simulink model "narwhale_3dof_dynamics_func"  (R2021b)
settings: Solver=VariableStepAuto  StartTime=0.0  StopTime=5  RelTol=1e-3
undefined symbols (not defined in the file or in its folder): X, Y, Z
libraries: sm_lib x20, nesl_utility x10
(part 2 of 2)

== matlab function narwhale_3dof_dynamics_func/NarWhale/MATLAB Function ==
  data: q1d input; ut output; q1v input; q1a input; q2d input; q2v input; q2a input; q3d input; q3v input; q3a input
function ut = fcn(q1d,q1v,q1a,q2d,q2v,q2a,q3d,q3v,q3a)

m1 = 3.0358
m2 = 2.0778
m3 = 1.4388
I1 = [0.00971694169       -0.00064648471      -0.01364762489;
      -0.00064648471        0.01128154665     -0.00136042243;
      -0.01364762489    -0.00136042243       0.01196416148];
I2 = [0.00247391072       -0.00003538205         -0.00217523776;
      -0.00003538205         0.03115417518       0.000038745;
      -0.00217523776       0.000038745         0.029417341];
I3 = [0.0016       0.00001724909   -0.00032435212;
      0.00001724909   0.0174       0.00000416776;
      -0.00032435212    0.00000416776       0.0164];

m = [m1 m2 m3]
I = cat(3,I1,I2,I3)
q = [q1d;q2d;q3d];
qd = [q1v;q2v ;q3v];
qdd = [q1a;q2a;q3a];
rho = [1;1;1];
%%
% parameters
    cm1 = [-43.29; -2.02; -88.16]./1000.0;
    cm2 = [162; -0.02; 8.59]./1000.0;
    cm3 = [-175.56; 0.06; -6.33]./1000.0;
    cm=cat(3,cm1,cm2,cm3);
    %find m
    Mt =zeros(3,3);
    Ct =zeros(3,3);
    Gt =zeros(3,1);
    ut =zeros(3,1);
    M = zeros(3,3,3);
    Hcm = zeros(4,4,3);
    Jwc = zeros(3,3,3);
    Jvc = zeros(3,3,3);
    % forwardkinematics
    h1= 275.99/1000.0; % lasted
    h2= 380.0/1000.0;
    l1= 20.0/1000.0;
    l2= 380.0/1000.0;
    l3= 268.23/1000.0;
    DH =[0   0   h1   0;
        l1 pi/2  0  pi/2;
        h2  0    0  -pi/2];
    
    Hne=[1 0  0  l2 ;
         0 1  0  0; 
         0 0  1  0;
         0 0  0  1];
    H1c1 = [1 0 0 cm1(1);
       0 1 0  cm1(2);
       0 0 1  cm1(3);
       0 0 0     1];
    H2c2 = [1 0 0 cm2(1);
            0 1 0 cm2(2);
            0 0 1 cm2(3);
            0 0 0    1];
    H3c3 = [1 0 0 cm3(1);
            0 1 0 cm3(2);
            0 0 1 cm3(3);
            0 0 0    1];
    m1 = m(1);
    m2 = m(2);
    m3 = m(3);
    g = 9.80665;

    q1 =q(1);
    q2 =q(2);
    q3 =q(3);
    q1d = qd(1);
    q2d = qd(2);
    q3d = qd(3);
    q1dd = qdd(1);
    q2dd = qdd(2);
    q3dd = qdd(3);
    H = forwardKinematics(q(1:3),rho,DH,Hne);
    Hcm(:,:,1) = H(:,:,1)*H1c1;
    Hcm(:,:,2) = H(:,:,2)*H2c2;
    Hcm(:,:,3) = H(:,:,3)*H3c3;
    S =@(P) [ 0   -P(3)  P(2);
              P(3)  0    -P(1);
             -P(2)  P(1)   0];
        
%         Jv_c1 = J(4:6,:,1)+S(H(1:3,1:3,1)*cm1).' * J(1:3,:,1);
%         Jv_c2 = J(4:6,:,2)+S(H(1:3,1:3,2)*cm2).' * J(1:3,:,2);
%         Jv_c3 = J(4:6,:,3)+S(H(1:3,1:3,3)*cm3).' * J(1:3,:,3);
    %Jacobian
    Jwc(:,:,1) = [0, 0, 0;
              0, 0, 0;
              1, 0, 0];
    Jwc(:,:,2) =[0,  sin(q1), 0;
             0, -cos(q1), 0;
             1,        0, 0];
    Jwc(:,:,3) =[0,  sin(q1),  sin(q1);
             0, -cos(q1), -cos(q1);
             1,        0,        0];
    Jvc(:,:,1) =[- cm1(2)*cos(q1) - cm1(1)*sin(q1), 0, 0;
               cm1(1)*cos(q1) - cm1(2)*sin(q1), 0, 0;
                                         0, 0, 0];
    Jvc(:,:,2) =[cm2(3)*cos(q1) - l1*sin(q1) + cm2(2)*cos(q2)*sin(q1) + cm2(1)*sin(q1)*sin(q2), -cos(q1)*(cm2(1)*cos(q2) - cm2(2)*sin(q2)), 0;
             l1*cos(q1) + cm2(3)*sin(q1) - cm2(2)*cos(q1)*cos(q2) - cm2(1)*cos(q1)*sin(q2), -sin(q1)*(cm2(1)*cos(q2) - cm2(2)*sin(q2)), 0;
                                                                                   0,          - cm2(2)*cos(q2) - cm2(1)*sin(q2), 0]
    Jvc(:,:,3) =[cm3(3)*cos(q1) - l1*sin(q1) - cm3(1)*cos(q2 + q3)*sin(q1) + cm3(2)*sin(q2 + q3)*sin(q1) + h2*sin(q1)*sin(q2), -cos(q1)*(cm3(2)*cos(q2 + q3) + cm3(1)*sin(q2 + q3) + h2*cos(q2)), -cos(q1)*(cm3(2)*cos(q2 + q3) + cm3(1)*sin(q2 + q3));
             l1*cos(q1) + cm3(3)*sin(q1) + cm3(1)*cos(q2 + q3)*cos(q1) - cm3(2)*sin(q2 + q3)*cos(q1) - h2*cos(q1)*sin(q2), -sin(q1)*(cm3(2)*cos(q2 + q3) + cm3(1)*sin(q2 + q3) + h2*cos(q2)), -sin(q1)*(cm3(2)*cos(q2 + q3) + cm3(1)*sin(q2 + q3));
                                                                                                                       0,            cm3(1)*cos(q2 + q3) - cm3(2)*sin(q2 + q3) - h2*sin(q2),            cm3(1)*cos(q2 + q3) - cm3(2)*sin(q2 + q3)];
 
    for j = 1:numel(rho)
            M(:,:,j) = (m(j)*(Jvc(:,:,j)')*Jvc(:,:,j)) + ((Jwc(:,:,j)')*Hcm(1:3,1:3,j)*I(:,:,j)*Hcm(1:3,1:3,j)'*Jwc(1:3,:,j));
    end
        sigmaM = M(:,:,1) + M(:,:,2) + M(:,:,3);
        Mt(:,:)=sigmaM;
        
        C = [0.5000*q3d*(cos(q2 + q3)*(I(2,1,3)*cos(q2 + q3) + I(1,1,3)*sin(q2 + q3)) + cos(q2 + q3)*(I(1,2,3)*cos(q2 + q3) - I(2,2,3)*sin(q2 + q3)) + sin(q2 + q3)*(I(1,1,3)*cos(q2 + q3) - I(2,1,3)*sin(q2 + q3)) - sin(q2 + q3)*(I(2,2,3)*cos(q2 + q3) + I(1,2,3)*sin(q2 + q3)) - 2*m3*(cm3(2)*cos(q2 + q3)*cos(q1) + cm3(1)*sin(q2 + q3)*cos(q1))*(l1*cos(q1) + cm3(3)*sin(q1) + cm3(1)*cos(q2 + q3)*cos(q1) - cm3(2)*sin(q2 + q3)*cos(q1) - h2*cos(q1)*sin(q2)) + 2*m3*(cm3(2)*cos(q2 + q3)*sin(q1) + cm3(1)*sin(q2 + q3)*sin(q1))*(cm3(3)*cos(q1) - l1*sin(q1) - cm3(1)*cos(q2 + q3)*sin(q1) + cm3(2)*sin(q2 + q3)*sin(q1) + h2*sin(q1)*sin(q2))) + 0.5000*q2d*(cos(q2 + q3)*(I(2,1,3)*cos(q2 + q3) + I(1,1,3)*sin(q2 + q3)) + cos(q2 + q3)*(I(1,2,3)*cos(q2 + q3) - I(2,2,3)*sin(q2 + q3)) + sin(q2 + q3)*(I(1,1,3)*cos(q2 + q3) - I(2,1,3)*sin(q2 + q3)) - sin(q2 + q3)*(I(2,2,3)*cos(q2 + q3) + I(1,2,3)*sin(q2 + q3)) - cos(q2)*(I(2,1,2)*cos(q2) + I(1,1,2)*sin(q2)) - cos(q2)*(I(1,2,2)*cos(q2) - I(2,2,2)*sin(q2)) - sin(q2)*(I(1,1,2)*cos(q2) - I(2,1,2)*sin(q2)) + sin(q2)*(I(2,2,2)*cos(q2) + I(1,2,2)*sin(q2)) + 2*m3*(cm3(2)*cos(q2 + q3)*sin(q1) + cm3(1)*sin(q2 + q3)*sin(q1) + h2*cos(q2)*sin(q1))*(cm3(3)*cos(q1) - l1*sin(q1) - cm3(1)*cos(q2 + q3)*sin(q1) + cm3(2)*sin(q2 + q3)*sin(q1) + h2*sin(q1)*sin(q2)) - 2*m2*(cm2(1)*cos(q1)*cos(q2) - cm2(2)*cos(q1)*sin(q2))*(l1*cos(q1) + cm2(3)*sin(q1) - cm2(2)*cos(q1)*cos(q2) - cm2(1)*cos(q1)*sin(q2)) - 2*m3*(cm3(2)*cos(q2 + q3)*cos(q1) + cm3(1)*sin(q2 + q3)*cos(q1) + h2*cos(q1)*cos(q2))*(l1*cos(q1) + cm3(3)*sin(q1) + cm3(1)*cos(q2 + q3)*cos(q1) - cm3(2)*sin(q2 + q3)*cos(q1) - h2*cos(q1)*sin(q2)) + 2*m2*(cm2(1)*cos(q2)*sin(q1) - cm2(2)*sin(q1)*sin(q2))*(cm2(3)*cos(q1) - l1*sin(q1) + cm2(2)*cos(q2)*sin(q1) + cm2(1)*sin(q1)*sin(q2))), 0.5000*q1d*(cos(q2 + q3)*(I(2,1,3)*cos(q2 + q3) + I(1,1,3)*sin(q2 + q3)) + cos(q2 + q3)*(I(1,2,3)*cos(q2 + q3) - I(2,2,3)*sin(q2 + q3)) + sin(q2 + q3)*(I(1,1,3)*cos(q2 + q3) - I(2,1,3)*sin(q2 + q3)) - sin(q2 + q3)*(I(2,2,3)*cos(q2 + q3) + I(1,2,3)*sin(q2 + q3)) - cos(q2)*(I(2,1,2)*cos(q2) + I(1,1,2)*sin(q2)) - cos(q2)*(I(1,2,2)*cos(q2) - I(2,2,2)*sin(q2)) - sin(q2)*(I(1,1,2)*cos(q2) - I(2,1,2)*sin(q2)) + sin(q2)*(I(2,2,2)*cos(q2) + I(1,2,2)*sin(q2)) + 2*m3*(cm3(2)*cos(q2 + q3)*sin(q1) + cm3(1)*sin(q2 + q3)*sin(q1) + h2*cos(q2)*sin(q1))*(cm3(3)*cos(q1) - l1*sin(q1) - cm3(1)*cos(q2 + q3)*sin(q1) + cm3(2)*sin(q2 + q3)*sin(q1) + h2*sin(q1)*sin(q2)) - 2*m2*(cm2(1)*cos(q1)*cos(q2) - cm2(2)*cos(q1)*sin(q2))*(l1*cos(q1) + cm2(3)*sin(q1) - cm2(2)*cos(q1)*cos(q2) - cm2(1)*cos(q1)*sin(q2)) - 2*m3*(cm3(2)*cos(q2 + q3)*cos(q1) + cm3(1)*sin(q2 + q3)*cos(q1) + h2*cos(q1)*cos(q2))*(l1*cos(q1) + cm3(3)*sin(q1) + cm3(1)*cos(q2 + q3)*cos(q1) - cm3(2)*sin(q2 + q3)*cos(q1) - h2*cos(q1)*sin(q2)) + 2*m2*(cm2(1)*cos(q2)*sin(q1) - cm2(2)*sin(q1)*sin(q2))*(cm2(3)*cos(q1) - l1*sin(q1) + cm2(2)*cos(q2)*sin(q1) + cm2(1)*sin(q1)*sin(q2))) - 0.5000*q3d*(2*sin(q1)*(cos(q2 + q3)*cos(q1)*(I(2,2,3)*cos(q2 + q3) + I(1,2,3)*sin(q2 + q3)) - cos(q2 + q3)*cos(q1)*(I(1,1,3)*cos(q2 + q3) - I(2,1,3)*sin(q2 + q3)) - sin(q1)*(I(1,3,3)*cos(q2 + q3) - I(2,3,3)*sin(q2 + q3)) + sin(q2 + q3)*cos(q1)*(I(2,1,3)*cos(q2 + q3) + I(1,1,3)*sin(q2 + q3)) + sin(q2 + q3)*cos(q1)*(I(1,2,3)*cos(q2 + q3) - I(2,2,3)*sin(q2 + q3))) - 2*cos(q1)*(cos(q1)*(I(1,3,3)*cos(q2 + q3) - I(2,3,3)*sin(q2 + q3)) + sin(q2 + q3)*sin(q1)*(I(2,1,3)*cos(q2 + q3) + I(1,1,3)*sin(q2 + q3)) + sin(q2 + q3)*sin(q1)*(I(1,2,3)*cos(q2 + q3) - I(2,2,3)*sin(q2 + q3)) - cos(q2 + q3)*sin(q1)*(I(1,1,3)*cos(q2 + q3) - I(2,1,3)*sin(q2 + q3)) + cos(q2 + q3)*sin(q1)*(I(2,2,3)*cos(q2 + q3) + I(1,2,3)*sin(q2 + q3))) - m3*sin(q1)*(cm3(2)*cos(q2 + q3) + cm3(1)*sin(q2 + q3))*(cm3(2)*cos(q2 + q3)*cos(q1) + cm3(1)*sin(q2 + q3)*cos(q1) + h2*cos(q1)*cos(q2)) + m3*cos(q1)*(cm3(2)*cos(q2 + q3) + cm3(1)*sin(q2 + q3))*(cm3(2)*cos(q2 + q3)*sin(q1) + cm3(1)*sin(q2 + q3)*sin(q1) + h2*cos(q2)*sin(q1)) - m3*sin(q1)*(cm3(2)*cos(q2 + q3)*cos(q1) + cm3(1)*sin(q2 + q3)*cos(q1))*(cm3(2)*cos(q2 + q3) + cm3(1)*sin(q2 + q3) + h2*cos(q2)) + m3*cos(q1)*(cm3(2)*cos(q2 + q3)*sin(q1) + cm3(1)*sin(q2 + q3)*sin(q1))*(cm3(2)*cos(q2 + q3) + cm3(1)*sin(q2 + q3) + h2*cos(q2)) + 2*m3*sin(q1)*(cm3(1)*cos(q2 + q3) - cm3(2)*sin(q2 + q3))*(l1*cos(q1) + cm3(3)*sin(q1) + cm3(1)*cos(q2 + q3)*cos(q1) - cm3(2)*sin(q2 + q3)*cos(q1) - h2*cos(q1)*sin(q2)) + 2*m3*cos(q1)*(cm3(1)*cos(q2 + q3) - cm3(2)*sin(q2 + q3))*(cm3(3)*cos(q1) - l1*sin(q1) - cm3(1)*cos(q2 + q3)*sin(q1) + cm3(2)*sin(q2 + q3)*sin(q1) + h2*sin(q1)*sin(q2))) + 0.5000*q2d*(2*sin(q1)*(cos(q1)*cos(q2)*(I(2,2,2)*cos(q2) + I(1,2,2)*sin(q2)) - cos(q1)*cos(q2)*(I(1,1,2)*cos(q2) - I(2,1,2)*sin(q2)) - sin(q1)*(I(2,3,2)*cos(q2) + I(1,3,2)*sin(q2)) + cos(q1)*sin(q2)*(I(2,1,2)*cos(q2) + I(1,1,2)*sin(q2)) + cos(q1)*sin(q2)*(I(1,2,2)*cos(q2) - I(2,2,2)*sin(q2))) - 2*cos(q1)*(cos(q1)*(I(2,3,2)*cos(q2) + I(1,3,2)*sin(q2)) - cos(q2)*sin(q1)*(I(1,1,2)*cos(q2) - I(2,1,2)*sin(q2)) + cos(q2)*sin(q1)*(I(2,2,2)*cos(q2) + I(1,2,2)*sin(q2)) + sin(q1)*sin(q2)*(I(2,1,2)*cos(q2) + I(1,1,2)*sin(q2)) + sin(q1)*sin(q2)*(I(1,2,2)*cos(q2) - I(2,2,2)*sin(q2))) - 2*sin(q1)*(cos(q2 + q3)*cos(q1)*(I(2,2,3)*cos(q2 + q3) + I(1,2,3)*sin(q2 + q3)) - cos(q2 + q3)*cos(q1)*(I(1,1,3)*cos(q2 + q3) - I(2,1,3)*sin(q2 + q3)) - sin(q1)*(I(1,3,3)*cos(q2 + q3) - I(2,3,3)*sin(q2 + q3)) + sin(q2 + q3)*cos(q1)*(I(2,1,3)*cos(q2 + q3) + I(1,1,3)*sin(q2 + q3)) + sin(q2 + q3)*cos(q1)*(I(1,2,3)*cos(q2 + q3) - I(2,2,3)*sin(q2 + q3))) + 2*cos(q1)*(cos(q1)*(I(1,3,3)*cos(q2 + q3) - I(2,3,3)*sin(q2 + q3)) + sin(q2 + q3)*sin(q1)*(I(2,1,3)*cos(q2 + q3) + I(1,1,3)*sin(q2 + q3)) + sin(q2 + q3)*sin(q1)*(I(1,2,3)*cos(q2 + q3) - I(2,2,3)*sin(q2 + q3)) - cos(q2 + q3)*sin(q1)*(I(1,1,3)*cos(q2 + q3) - I(2,1,3)*sin(q2 + q3)) + cos(q2 + q3)*sin(q1)*(I(2,2,3)*cos(q2 + q3) + I(1,2,3)*sin(q2 + q3))) - 2*m3*cos(q1)*(cm3(2)*cos(q2 + q3)*sin(q1) + cm3(1)*sin(q2 + q3)*sin(q1) + h2*cos(q2)*sin(q1))*(cm3(2)*cos(q2 + q3) + cm3(1)*sin(q2 + q3) + h2*cos(q2)) + 2*m3*sin(q1)*(cm3(2)*sin(q2 + q3) - cm3(1)*cos(q2 + q3) + h2*sin(q2))*(l1*cos(q1) + cm3(3)*sin(q1) + cm3(1)*cos(q2 + q3)*cos(q1) - cm3(2)*sin(q2 + q3)*cos(q1) - h2*cos(q1)*sin(q2)) + 2*m3*cos(q1)*(cm3(2)*sin(q2 + q3) - cm3(1)*cos(q2 + q3) + h2*sin(q2))*(cm3(3)*cos(q1) - l1*sin(q1) - cm3(1)*cos(q2 + q3)*sin(q1) + cm3(2)*sin(q2 + q3)*sin(q1) + h2*sin(q1)*sin(q2)) + 2*m2*sin(q1)*(cm2(1)*cos(q1)*cos(q2) - cm2(2)*cos(q1)*sin(q2))*(cm2(1)*cos(q2) - cm2(2)*sin(q2)) - 2*m2*cos(q1)*(cm2(1)*cos(q2)*sin(q1) - cm2(2)*sin(q1)*sin(q2))*(cm2(1)*cos(q2) - cm2(2)*sin(q2)) + 2*m2*sin(q1)*(cm2(2)*cos(q2) + cm2(1)*sin(q2))*(l1*cos(q1) + cm2(3)*sin(q1) - cm2(2)*cos(q1)*cos(q2) - cm2(1)*cos(q1)*sin(q2)) + 2*m3*sin(q1)*(cm3(2)*cos(q2 + q3)*cos(q1) + cm3(1)*sin(q2 + q3)*cos(q1) + h2*cos(q1)*cos(q2))*(cm3(2)*cos(q2 + q3) + cm3(1)*sin(q2 + q3) + h2*cos(q2)) + 2*m2*cos(q1)*(cm2(2)*cos(q2) + cm2(1)*sin(q2))*(cm2(3)*cos(q1) - l1*sin(q1) + cm2(2)*cos(q2)*sin(q1) + cm2(1)*sin(q1)*sin(q2))), 0.5000*q1d*(cos(q2 + q3)*(I(2,1,3)*cos(q2 + q3) + I(1,1,3)*sin(q2 + q3)) + cos(q2 + q3)*(I(1,2,3)*cos(q2 + q3) - I(2,2,3)*sin(q2 + q3)) + sin(q2 + q3)*(I(1,1,3)*cos(q2 + q3) - I(2,1,3)*sin(q2 + q3)) - sin(q2 + q3)*(I(2,2,3)*cos(q2 + q3) + I(1,2,3)*sin(q2 + q3)) - 2*m3*(cm3(2)*cos(q2 + q3)*cos(q1) + cm3(1)*sin(q2 + q3)*cos(q1))*(l1*cos(q1) + cm3(3)*sin(q1) + cm3(1)*cos(q2 + q3)*cos(q1) - cm3(2)*sin(q2 + q3)*cos(q1) - h2*cos(q1)*sin(q2)) + 2*m3*(cm3(2)*cos(q2 + q3)*sin(q1) + cm3(1)*sin(q2 + q3)*sin(q1))*(cm3(3)*cos(q1) - l1*sin(q1) - cm3(1)*cos(q2 + q3)*sin(q1) + cm3(2)*sin(q2 + q3)*sin(q1) + h2*sin(q1)*sin(q2))) - 0.5000*q2d*(2*sin(q1)*(cos(q2 + q3)*cos(q1)*(I(2,2,3)*cos(q2 + q3) + I(1,2,3)*sin(q2 + q3)) - cos(q2 + q3)*cos(q1)*(I(1,1,3)*cos(q2 + q3) - I(2,1,3)*sin(q2 + q3)) - sin(q1)*(I(1,3,3)*cos(q2 + q3) - I(2,3,3)*sin(q2 + q3)) + sin(q2 + q3)*cos(q1)*(I(2,1,3)*cos(q2 + q3) + I(1,1,3)*sin(q2 + q3)) + sin(q2 + q3)*cos(q1)*(I(1,2,3)*cos(q2 + q3) - I(2,2,3)*sin(q2 + q3))) - 2*cos(q1)*(cos(q1)*(I(1,3,3)*cos(q2 + q3) - I(2,3,3)*sin(q2 + q3)) + sin(q2 + q3)*sin(q1)*(I(2,1,3)*cos(q2 + q3) + I(1,1,3)*sin(q2 + q3)) + sin(q2 + q3)*sin(q1)*(I(1,2,3)*cos(q2 + q3) - I(2,2,3)*sin(q2 + q3)) - cos(q2 + q3)*sin(q1)*(I(1,1,3)*cos(q2 + q3) - I(2,1,3)*sin(q2 + q3)) + cos(q2 + q3)*sin(q1)*(I(2,2,3)*cos(q2 + q3) + I(1,2,3)*sin(q2 + q3))) - m3*sin(q1)*(cm3(2)*cos(q2 + q3) + cm3(1)*sin(q2 + q3))*(cm3(2)*cos(q2 + q3)*cos(q1) + cm3(1)*sin(q2 + q3)*cos(q1) + h2*cos(q1)*cos(q2)) + m3*cos(q1)*(cm3(2)*cos(q2 + q3) + cm3(1)*sin(q2 + q3))*(cm3(2)*cos(q2 + q3)*sin(q1) + cm3(1)*sin(q2 + q3)*sin(q1) + h2*cos(q2)*sin(q1)) - m3*sin(q1)*(cm3(2)*cos(q2 + q3)*cos(q1) + cm3(1)*sin(q2 + q3)*cos(q1))*(cm3(2)*cos(q2 + q3) + cm3(1)*sin(q2 + q3) + h2*cos(q2)) + m3*cos(q1)*(cm3(2)*cos(q2 + q3)*sin(q1) + cm3(1)*sin(q2 + q3)*sin(q1))*(cm3(2)*cos(q2 + q3) + cm3(1)*sin(q2 + q3) + h2*cos(q2)) + 2*m3*sin(q1)*(cm3(1)*cos(q2 + q3) - cm3(2)*sin(q2 + q3))*(l1*cos(q1) + cm3(3)*sin(q1) + cm3(1)*cos(q2 + q3)*cos(q1) - cm3(2)*sin(q2 + q3)*cos(q1) - h2*cos(q1)*sin(q2)) + 2*m3*cos(q1)*(cm3(1)*cos(q2 + q3) - cm3(2)*sin(q2 + q3))*(cm3(3)*cos(q1) - l1*sin(q1) - cm3(1)*cos(q2 + q3)*sin(q1) + cm3(2)*sin(q2 + q3)*sin(q1) + h2*sin(q1)*sin(q2))) - 0.5000*q3d*(2*sin(q1)*(cos(q2 + q3)*cos(q1)*(I(2,2,3)*cos(q2 + q3) + I(1,2,3)*sin(q2 + q3)) - cos(q2 + q3)*cos(q1)*(I(1,1,3)*cos(q2 + q3) - I(2,1,3)*sin(q2 + q3)) - sin(q1)*(I(1,3,3)*cos(q2 + q3) - I(2,3,3)*sin(q2 + q3)) + sin(q2 + q3)*cos(q1)*(I(2,1,3)*cos(q2 + q3) + I(1,1,3)*sin(q2 + q3)) + sin(q2 + q3)*cos(q1)*(I(1,2,3)*cos(q2 + q3) - I(2,2,3)*sin(q2 + q3))) - 2*cos(q1)*(cos(q1)*(I(1,3,3)*cos(q2 + q3) - I(2,3,3)*sin(q2 + q3)) + sin(q2 + q3)*sin(q1)*(I(2,1,3)*cos(q2 + q3) + I(1,1,3)*sin(q2 + q3)) + sin(q2 + q3)*sin(q1)*(I(1,2,3)*cos(q2 + q3) - I(2,2,3)*sin(q2 + q3)) - cos(q2 + q3)*sin(q1)*(I(1,1,3)*cos(q2 + q3) - I(2,1,3)*sin(q2 + q3)) + cos(q2 + q3)*sin(q1)*(I(2,2,3)*cos(q2 + q3) + I(1,2,3)*sin(q2 + q3))) + 2*m3*sin(q1)*(cm3(1)*cos(q2 + q3) - cm3(2)*sin(q2 + q3))*(l1*cos(q1) + cm3(3)*sin(q1) + cm3(1)*cos(q2 + q3)*cos(q1) - cm3(2)*sin(q2 + q3)*cos(q1) - h2*cos(q1)*sin(q2)) + 2*m3*cos(q1)*(cm3(1)*cos(q2 + q3) - cm3(2)*sin(q2 + q3))*(cm3(3)*cos(q1) - l1*sin(q1) - cm3(1)*cos(q2 + q3)*sin(q1) + cm3(2)*sin(q2 + q3)*sin(q1) + h2*sin(q1)*sin(q2)) - 2*m3*sin(q1)*(cm3(2)*cos(q2 + q3) + cm3(1)*sin(q2 + q3))*(cm3(2)*cos(q2 + q3)*cos(q1) + cm3(1)*sin(q2 + q3)*cos(q1)) + 2*m3*cos(q1)*(cm3(2)*cos(q2 + q3)*sin(q1) + cm3(1)*sin(q2 + q3)*sin(q1))*(cm3(2)*cos(q2 + q3) + cm3(1)*sin(q2 + q3)));
                                                          - 0.5000*q1d*(cos(q2 + q3)*(I(2,1,3)*cos(q2 + q3) + I(1,1,3)*sin(q2 + q3)) + cos(q2 + q3)*(I(1,2,3)*cos(q2 + q3) - I(2,2,3)*sin(q2 + q3)) + sin(q2 + q3)*(I(1,1,3)*cos(q2 + q3) - I(2,1,3)*sin(q2 + q3)) - sin(q2 + q3)*(I(2,2,3)*cos(q2 + q3) + I(1,2,3)*sin(q2 + q3)) - cos(q2)*(I(2,1,2)*cos(q2) + I(1,1,2)*sin(q2)) - cos(q2)*(I(1,2,2)*cos(q2) - I(2,2,2)*sin(q2)) - sin(q2)*(I(1,1,2)*cos(q2) - I(2,1,2)*sin(q2)) + sin(q2)*(I(2,2,2)*cos(q2) + I(1,2,2)*sin(q2)) + 2*m3*(cm3(2)*cos(q2 + q3)*sin(q1) + cm3(1)*sin(q2 + q3)*sin(q1) + h2*cos(q2)*sin(q1))*(cm3(3)*cos(q1) - l1*sin(q1) - cm3(1)*cos(q2 + q3)*sin(q1) + cm3(2)*sin(q2 + q3)*sin(q1) + h2*sin(q1)*sin(q2)) - 2*m2*(cm2(1)*cos(q1)*cos(q2) - cm2(2)*cos(q1)*sin(q2))*(l1*cos(q1) + cm2(3)*sin(q1) - cm2(2)*cos(q1)*cos(q2) - cm2(1)*cos(q1)*sin(q2)) - 2*m3*(cm3(2)*cos(q2 + q3)*cos(q1) + cm3(1)*sin(q2 + q3)*cos(q1) + h2*cos(q1)*cos(q2))*(l1*cos(q1) + cm3(3)*sin(q1) + cm3(1)*cos(q2 + q3)*cos(q1) - cm3(2)*sin(q2 + q3)*cos(q1) - h2*cos(q1)*sin(q2)) + 2*m2*(cm2(1)*cos(q2)*sin(q1) - cm2(2)*sin(q1)*sin(q2))*(cm2(3)*cos(q1) - l1*sin(q1) + cm2(2)*cos(q2)*sin(q1) + cm2(1)*sin(q1)*sin(q2))) - 0.5000*q3d*(m3*sin(q1)*(cm3(2)*cos(q2 + q3) + cm3(1)*sin(q2 + q3))*(cm3(2)*cos(q2 + q3)*cos(q1) + cm3(1)*sin(q2 + q3)*cos(q1) + h2*cos(q1)*cos(q2)) - m3*cos(q1)*(cm3(2)*cos(q2 + q3) + cm3(1)*sin(q2 + q3))*(cm3(2)*cos(q2 + q3)*sin(q1) + cm3(1)*sin(q2 + q3)*sin(q1) + h2*cos(q2)*sin(q1)) - m3*sin(q1)*(cm3(2)*cos(q2 + q3)*cos(q1) + cm3(1)*sin(q2 + q3)*cos(q1))*(cm3(2)*cos(q2 + q3) + cm3(1)*sin(q2 + q3) + h2*cos(q2)) + m3*cos(q1)*(cm3(2)*cos(q2 + q3)*sin(q1) + cm3(1)*sin(q2 + q3)*sin(q1))*(cm3(2)*cos(q2 + q3) + cm3(1)*sin(q2 + q3) + h2*cos(q2))),                                                                                                                                                                                                                                                                                                                                                                                                                                                                                                                                                                                                                                                                                                                                                                                                                                                                                                                                                                                                                                                                                                                                                                                                                                                                                                                                                                                                                                                                                                                                                                                                                                                                                                                                                                                                                                                                                           0.5000*q3d*(cos(q1)*(I(3,2,3)*cos(q2 + q3)*sin(q1)*(cos(q1)^2 + sin(q1)^2) + I(3,1,3)*sin(q2 + q3)*sin(q1)*(cos(q1)^2 + sin(q1)^2)) - sin(q1)*(I(3,1,3)*sin(q2 + q3)*cos(q1)*(cos(q1)^2 + sin(q1)^2) + I(3,2,3)*cos(q2 + q3)*cos(q1)*(cos(q1)^2 + sin(q1)^2)) + 2*m3*(cm3(2)*cos(q2 + q3) + cm3(1)*sin(q2 + q3))*(cm3(2)*sin(q2 + q3) - cm3(1)*cos(q2 + q3) + h2*sin(q2)) + 2*m3*cos(q1)^2*(cm3(1)*cos(q2 + q3) - cm3(2)*sin(q2 + q3))*(cm3(2)*cos(q2 + q3) + cm3(1)*sin(q2 + q3) + h2*cos(q2)) + 2*m3*sin(q1)^2*(cm3(1)*cos(q2 + q3) - cm3(2)*sin(q2 + q3))*(cm3(2)*cos(q2 + q3) + cm3(1)*sin(q2 + q3) + h2*cos(q2))) - 0.5000*q2d*(sin(q1)*(I(3,1,2)*cos(q1)*cos(q2)*(cos(q1)^2 + sin(q1)^2) - I(3,2,2)*cos(q1)*sin(q2)*(cos(q1)^2 + sin(q1)^2)) - cos(q1)*(I(3,1,2)*cos(q2)*sin(q1)*(cos(q1)^2 + sin(q1)^2) - I(3,2,2)*sin(q1)*sin(q2)*(cos(q1)^2 + sin(q1)^2)) + sin(q1)*(I(3,1,3)*sin(q2 + q3)*cos(q1)*(cos(q1)^2 + sin(q1)^2) + I(3,2,3)*cos(q2 + q3)*cos(q1)*(cos(q1)^2 + sin(q1)^2)) - cos(q1)*(I(3,2,3)*cos(q2 + q3)*sin(q1)*(cos(q1)^2 + sin(q1)^2) + I(3,1,3)*sin(q2 + q3)*sin(q1)*(cos(q1)^2 + sin(q1)^2)) - 2*m2*(cm2(2)*cos(q2) + cm2(1)*sin(q2))*(cm2(1)*cos(q2) - cm2(2)*sin(q2)) - 2*m3*(cm3(2)*cos(q2 + q3) + cm3(1)*sin(q2 + q3) + h2*cos(q2))*(cm3(2)*sin(q2 + q3) - cm3(1)*cos(q2 + q3) + h2*sin(q2)) + 2*m2*cos(q1)^2*(cm2(2)*cos(q2) + cm2(1)*sin(q2))*(cm2(1)*cos(q2) - cm2(2)*sin(q2)) + 2*m2*sin(q1)^2*(cm2(2)*cos(q2) + cm2(1)*sin(q2))*(cm2(1)*cos(q2) - cm2(2)*sin(q2)) + 2*m3*cos(q1)^2*(cm3(2)*cos(q2 + q3) + cm3(1)*sin(q2 + q3) + h2*cos(q2))*(cm3(2)*sin(q2 + q3) - cm3(1)*cos(q2 + q3) + h2*sin(q2)) + 2*m3*sin(q1)^2*(cm3(2)*cos(q2 + q3) + cm3(1)*sin(q2 + q3) + h2*cos(q2))*(cm3(2)*sin(q2 + q3) - cm3(1)*cos(q2 + q3) + h2*sin(q2))) - 0.5000*q1d*(sin(q1)*(cos(q1)*cos(q2)*(I(2,2,2)*cos(q2) + I(1,2,2)*sin(q2)) - cos(q1)*cos(q2)*(I(1,1,2)*cos(q2) - I(2,1,2)*sin(q2)) - sin(q1)*(I(2,3,2)*cos(q2) + I(1,3,2)*sin(q2)) + cos(q1)*sin(q2)*(I(2,1,2)*cos(q2) + I(1,1,2)*sin(q2)) + cos(q1)*sin(q2)*(I(1,2,2)*cos(q2) - I(2,2,2)*sin(q2))) - cos(q1)*(cos(q1)*(I(2,3,2)*cos(q2) + I(1,3,2)*sin(q2)) - cos(q2)*sin(q1)*(I(1,1,2)*cos(q2) - I(2,1,2)*sin(q2)) + cos(q2)*sin(q1)*(I(2,2,2)*cos(q2) + I(1,2,2)*sin(q2)) + sin(q1)*sin(q2)*(I(2,1,2)*cos(q2) + I(1,1,2)*sin(q2)) + sin(q1)*sin(q2)*(I(1,2,2)*cos(q2) - I(2,2,2)*sin(q2))) - sin(q1)*(cos(q2 + q3)*cos(q1)*(I(2,2,3)*cos(q2 + q3) + I(1,2,3)*sin(q2 + q3)) - cos(q2 + q3)*cos(q1)*(I(1,1,3)*cos(q2 + q3) - I(2,1,3)*sin(q2 + q3)) - sin(q1)*(I(1,3,3)*cos(q2 + q3) - I(2,3,3)*sin(q2 + q3)) + sin(q2 + q3)*cos(q1)*(I(2,1,3)*cos(q2 + q3) + I(1,1,3)*sin(q2 + q3)) + sin(q2 + q3)*cos(q1)*(I(1,2,3)*cos(q2 + q3) - I(2,2,3)*sin(q2 + q3))) + cos(q1)*(cos(q1)*(I(1,3,3)*cos(q2 + q3) - I(2,3,3)*sin(q2 + q3)) + sin(q2 + q3)*sin(q1)*(I(2,1,3)*cos(q2 + q3) + I(1,1,3)*sin(q2 + q3)) + sin(q2 + q3)*sin(q1)*(I(1,2,3)*cos(q2 + q3) - I(2,2,3)*sin(q2 + q3)) - cos(q2 + q3)*sin(q1)*(I(1,1,3)*cos(q2 + q3) - I(2,1,3)*sin(q2 + q3)) + cos(q2 + q3)*sin(q1)*(I(2,2,3)*cos(q2 + q3) + I(1,2,3)*sin(q2 + q3))) - I(3,1,3)*cos(q2 + q3)*(cos(q1)^2 + sin(q1)^2) + I(3,2,3)*sin(q2 + q3)*(cos(q1)^2 + sin(q1)^2) + I(3,2,2)*cos(q2)*(cos(q1)^2 + sin(q1)^2) + I(3,1,2)*sin(q2)*(cos(q1)^2 + sin(q1)^2)),                                                                                                                                                                                                                                                                                                                                                                                                                                                                                                                                                                                                                                                                                                                                                                                                                                                                                                                     0.5000*q1d*(sin(q1)*(cos(q2 + q3)*cos(q1)*(I(2,2,3)*cos(q2 + q3) + I(1,2,3)*sin(q2 + q3)) - cos(q2 + q3)*cos(q1)*(I(1,1,3)*cos(q2 + q3) - I(2,1,3)*sin(q2 + q3)) - sin(q1)*(I(1,3,3)*cos(q2 + q3) - I(2,3,3)*sin(q2 + q3)) + sin(q2 + q3)*cos(q1)*(I(2,1,3)*cos(q2 + q3) + I(1,1,3)*sin(q2 + q3)) + sin(q2 + q3)*cos(q1)*(I(1,2,3)*cos(q2 + q3) - I(2,2,3)*sin(q2 + q3))) - cos(q1)*(cos(q1)*(I(1,3,3)*cos(q2 + q3) - I(2,3,3)*sin(q2 + q3)) + sin(q2 + q3)*sin(q1)*(I(2,1,3)*cos(q2 + q3) + I(1,1,3)*sin(q2 + q3)) + sin(q2 + q3)*sin(q1)*(I(1,2,3)*cos(q2 + q3) - I(2,2,3)*sin(q2 + q3)) - cos(q2 + q3)*sin(q1)*(I(1,1,3)*cos(q2 + q3) - I(2,1,3)*sin(q2 + q3)) + cos(q2 + q3)*sin(q1)*(I(2,2,3)*cos(q2 + q3) + I(1,2,3)*sin(q2 + q3))) + I(3,1,3)*cos(q2 + q3)*(cos(q1)^2 + sin(q1)^2) - I(3,2,3)*sin(q2 + q3)*(cos(q1)^2 + sin(q1)^2) - m3*sin(q1)*(cm3(2)*cos(q2 + q3) + cm3(1)*sin(q2 + q3))*(cm3(2)*cos(q2 + q3)*cos(q1) + cm3(1)*sin(q2 + q3)*cos(q1) + h2*cos(q1)*cos(q2)) + m3*cos(q1)*(cm3(2)*cos(q2 + q3) + cm3(1)*sin(q2 + q3))*(cm3(2)*cos(q2 + q3)*sin(q1) + cm3(1)*sin(q2 + q3)*sin(q1) + h2*cos(q2)*sin(q1)) + m3*sin(q1)*(cm3(2)*cos(q2 + q3)*cos(q1) + cm3(1)*sin(q2 + q3)*cos(q1))*(cm3(2)*cos(q2 + q3) + cm3(1)*sin(q2 + q3) + h2*cos(q2)) - m3*cos(q1)*(cm3(2)*cos(q2 + q3)*sin(q1) + cm3(1)*sin(q2 + q3)*sin(q1))*(cm3(2)*cos(q2 + q3) + cm3(1)*sin(q2 + q3) + h2*cos(q2))) + 0.5000*q2d*(cos(q1)*(I(3,2,3)*cos(q2 + q3)*sin(q1)*(cos(q1)^2 + sin(q1)^2) + I(3,1,3)*sin(q2 + q3)*sin(q1)*(cos(q1)^2 + sin(q1)^2)) - sin(q1)*(I(3,1,3)*sin(q2 + q3)*cos(q1)*(cos(q1)^2 + sin(q1)^2) + I(3,2,3)*cos(q2 + q3)*cos(q1)*(cos(q1)^2 + sin(q1)^2)) + 2*m3*(cm3(2)*cos(q2 + q3) + cm3(1)*sin(q2 + q3))*(cm3(2)*sin(q2 + q3) - cm3(1)*cos(q2 + q3) + h2*sin(q2)) + 2*m3*cos(q1)^2*(cm3(1)*cos(q2 + q3) - cm3(2)*sin(q2 + q3))*(cm3(2)*cos(q2 + q3) + cm3(1)*sin(q2 + q3) + h2*cos(q2)) + 2*m3*sin(q1)^2*(cm3(1)*cos(q2 + q3) - cm3(2)*sin(q2 + q3))*(cm3(2)*cos(q2 + q3) + cm3(1)*sin(q2 + q3) + h2*cos(q2))) + 0.5000*q3d*(cos(q1)*(I(3,2,3)*cos(q2 + q3)*sin(q1)*(cos(q1)^2 + sin(q1)^2) + I(3,1,3)*sin(q2 + q3)*sin(q1)*(cos(q1)^2 + sin(q1)^2)) - sin(q1)*(I(3,1,3)*sin(q2 + q3)*cos(q1)*(cos(q1)^2 + sin(q1)^2) + I(3,2,3)*cos(q2 + q3)*cos(q1)*(cos(q1)^2 + sin(q1)^2)) + 2*m3*(cm3(2)*cos(q2 + q3) + cm3(1)*sin(q2 + q3))*(cm3(2)*sin(q2 + q3) - cm3(1)*cos(q2 + q3) + h2*sin(q2)) + 2*m3*cos(q1)^2*(cm3(1)*cos(q2 + q3) - cm3(2)*sin(q2 + q3))*(cm3(2)*cos(q2 + q3) + cm3(1)*sin(q2 + q3) + h2*cos(q2)) + 2*m3*sin(q1)^2*(cm3(1)*cos(q2 + q3) - cm3(2)*sin(q2 + q3))*(cm3(2)*cos(q2 + q3) + cm3(1)*sin(q2 + q3) + h2*cos(q2)));
                                                                                                                                                                                                                                                                                                                                                                                                                                                                                                                                            0.5000*q2d*(m3*sin(q1)*(cm3(2)*cos(q2 + q3) + cm3(1)*sin(q2 + q3))*(cm3(2)*cos(q2 + q3)*cos(q1) + cm3(1)*sin(q2 + q3)*cos(q1) + h2*cos(q1)*cos(q2)) - m3*cos(q1)*(cm3(2)*cos(q2 + q3) + cm3(1)*sin(q2 + q3))*(cm3(2)*cos(q2 + q3)*sin(q1) + cm3(1)*sin(q2 + q3)*sin(q1) + h2*cos(q2)*sin(q1)) - m3*sin(q1)*(cm3(2)*cos(q2 + q3)*cos(q1) + cm3(1)*sin(q2 + q3)*cos(q1))*(cm3(2)*cos(q2 + q3) + cm3(1)*sin(q2 + q3) + h2*cos(q2)) + m3*cos(q1)*(cm3(2)*cos(q2 + q3)*sin(q1) + cm3(1)*sin(q2 + q3)*sin(q1))*(cm3(2)*cos(q2 + q3) + cm3(1)*sin(q2 + q3) + h2*cos(q2))) - 0.5000*q1d*(cos(q2 + q3)*(I(2,1,3)*cos(q2 + q3) + I(1,1,3)*sin(q2 + q3)) + cos(q2 + q3)*(I(1,2,3)*cos(q2 + q3) - I(2,2,3)*sin(q2 + q3)) + sin(q2 + q3)*(I(1,1,3)*cos(q2 + q3) - I(2,1,3)*sin(q2 + q3)) - sin(q2 + q3)*(I(2,2,3)*cos(q2 + q3) + I(1,2,3)*sin(q2 + q3)) - 2*m3*(cm3(2)*cos(q2 + q3)*cos(q1) + cm3(1)*sin(q2 + q3)*cos(q1))*(l1*cos(q1) + cm3(3)*sin(q1) + cm3(1)*cos(q2 + q3)*cos(q1) - cm3(2)*sin(q2 + q3)*cos(q1) - h2*cos(q1)*sin(q2)) + 2*m3*(cm3(2)*cos(q2 + q3)*sin(q1) + cm3(1)*sin(q2 + q3)*sin(q1))*(cm3(3)*cos(q1) - l1*sin(q1) - cm3(1)*cos(q2 + q3)*sin(q1) + cm3(2)*sin(q2 + q3)*sin(q1) + h2*sin(q1)*sin(q2))),                                                                                                                                                                                                                                                                                                                                                                                                                                                                                                                                                                                                                                                                                                                                                                                                                                                                                                                                                                                                                                                                                                                                                                                                                                                                                                                                                                                                                                                                                                                                                                                                                                                                                                                                                                                                                                                                                                                                                                                                                                                                                                                                                                                                                                                                                                                                                                                                                                                                                                          0.5000*q1d*(sin(q1)*(cos(q2 + q3)*cos(q1)*(I(2,2,3)*cos(q2 + q3) + I(1,2,3)*sin(q2 + q3)) - cos(q2 + q3)*cos(q1)*(I(1,1,3)*cos(q2 + q3) - I(2,1,3)*sin(q2 + q3)) - sin(q1)*(I(1,3,3)*cos(q2 + q3) - I(2,3,3)*sin(q2 + q3)) + sin(q2 + q3)*cos(q1)*(I(2,1,3)*cos(q2 + q3) + I(1,1,3)*sin(q2 + q3)) + sin(q2 + q3)*cos(q1)*(I(1,2,3)*cos(q2 + q3) - I(2,2,3)*sin(q2 + q3))) - cos(q1)*(cos(q1)*(I(1,3,3)*cos(q2 + q3) - I(2,3,3)*sin(q2 + q3)) + sin(q2 + q3)*sin(q1)*(I(2,1,3)*cos(q2 + q3) + I(1,1,3)*sin(q2 + q3)) + sin(q2 + q3)*sin(q1)*(I(1,2,3)*cos(q2 + q3) - I(2,2,3)*sin(q2 + q3)) - cos(q2 + q3)*sin(q1)*(I(1,1,3)*cos(q2 + q3) - I(2,1,3)*sin(q2 + q3)) + cos(q2 + q3)*sin(q1)*(I(2,2,3)*cos(q2 + q3) + I(1,2,3)*sin(q2 + q3))) + I(3,1,3)*cos(q2 + q3)*(cos(q1)^2 + sin(q1)^2) - I(3,2,3)*sin(q2 + q3)*(cos(q1)^2 + sin(q1)^2) + m3*sin(q1)*(cm3(2)*cos(q2 + q3) + cm3(1)*sin(q2 + q3))*(cm3(2)*cos(q2 + q3)*cos(q1) + cm3(1)*sin(q2 + q3)*cos(q1) + h2*cos(q1)*cos(q2)) - m3*cos(q1)*(cm3(2)*cos(q2 + q3) + cm3(1)*sin(q2 + q3))*(cm3(2)*cos(q2 + q3)*sin(q1) + cm3(1)*sin(q2 + q3)*sin(q1) + h2*cos(q2)*sin(q1)) - m3*sin(q1)*(cm3(2)*cos(q2 + q3)*cos(q1) + cm3(1)*sin(q2 + q3)*cos(q1))*(cm3(2)*cos(q2 + q3) + cm3(1)*sin(q2 + q3) + h2*cos(q2)) + m3*cos(q1)*(cm3(2)*cos(q2 + q3)*sin(q1) + cm3(1)*sin(q2 + q3)*sin(q1))*(cm3(2)*cos(q2 + q3) + cm3(1)*sin(q2 + q3) + h2*cos(q2))) - 0.5000*q2d*(sin(q1)*(I(3,1,3)*sin(q2 + q3)*cos(q1)*(cos(q1)^2 + sin(q1)^2) + I(3,2,3)*cos(q2 + q3)*cos(q1)*(cos(q1)^2 + sin(q1)^2)) - cos(q1)*(I(3,2,3)*cos(q2 + q3)*sin(q1)*(cos(q1)^2 + sin(q1)^2) + I(3,1,3)*sin(q2 + q3)*sin(q1)*(cos(q1)^2 + sin(q1)^2)) + 2*m3*(cm3(1)*cos(q2 + q3) - cm3(2)*sin(q2 + q3))*(cm3(2)*cos(q2 + q3) + cm3(1)*sin(q2 + q3) + h2*cos(q2)) + 2*m3*cos(q1)^2*(cm3(2)*cos(q2 + q3) + cm3(1)*sin(q2 + q3))*(cm3(2)*sin(q2 + q3) - cm3(1)*cos(q2 + q3) + h2*sin(q2)) + 2*m3*sin(q1)^2*(cm3(2)*cos(q2 + q3) + cm3(1)*sin(q2 + q3))*(cm3(2)*sin(q2 + q3) - cm3(1)*cos(q2 + q3) + h2*sin(q2))) + 0.5000*q3d*(cos(q1)*(I(3,2,3)*cos(q2 + q3)*sin(q1)*(cos(q1)^2 + sin(q1)^2) + I(3,1,3)*sin(q2 + q3)*sin(q1)*(cos(q1)^2 + sin(q1)^2)) - sin(q1)*(I(3,1,3)*sin(q2 + q3)*cos(q1)*(cos(q1)^2 + sin(q1)^2) + I(3,2,3)*cos(q2 + q3)*cos(q1)*(cos(q1)^2 + sin(q1)^2)) - 2*m3*(cm3(2)*cos(q2 + q3) + cm3(1)*sin(q2 + q3))*(cm3(1)*cos(q2 + q3) - cm3(2)*sin(q2 + q3)) + 2*m3*cos(q1)^2*(cm3(2)*cos(q2 + q3) + cm3(1)*sin(q2 + q3))*(cm3(1)*cos(q2 + q3) - cm3(2)*sin(q2 + q3)) + 2*m3*sin(q1)^2*(cm3(2)*cos(q2 + q3) + cm3(1)*sin(q2 + q3))*(cm3(1)*cos(q2 + q3) - cm3(2)*sin(q2 + q3))),                                                                                                                                                                                                                                                                                                                                                                                                                                                                                                                                                                                                                                                                                                                                                                                                                                                                                                                                                                                                                                                                                                                                                                                                                                                                                                                                                                                                                                                                                                                           0.5000*q2d*(cos(q1)*(I(3,2,3)*cos(q2 + q3)*sin(q1)*(cos(q1)^2 + sin(q1)^2) + I(3,1,3)*sin(q2 + q3)*sin(q1)*(cos(q1)^2 + sin(q1)^2)) - sin(q1)*(I(3,1,3)*sin(q2 + q3)*cos(q1)*(cos(q1)^2 + sin(q1)^2) + I(3,2,3)*cos(q2 + q3)*cos(q1)*(cos(q1)^2 + sin(q1)^2)) - 2*m3*(cm3(2)*cos(q2 + q3) + cm3(1)*sin(q2 + q3))*(cm3(1)*cos(q2 + q3) - cm3(2)*sin(q2 + q3)) + 2*m3*cos(q1)^2*(cm3(2)*cos(q2 + q3) + cm3(1)*sin(q2 + q3))*(cm3(1)*cos(q2 + q3) - cm3(2)*sin(q2 + q3)) + 2*m3*sin(q1)^2*(cm3(2)*cos(q2 + q3) + cm3(1)*sin(q2 + q3))*(cm3(1)*cos(q2 + q3) - cm3(2)*sin(q2 + q3))) + 0.5000*q3d*(cos(q1)*(I(3,2,3)*cos(q2 + q3)*sin(q1)*(cos(q1)^2 + sin(q1)^2) + I(3,1,3)*sin(q2 + q3)*sin(q1)*(cos(q1)^2 + sin(q1)^2)) - sin(q1)*(I(3,1,3)*sin(q2 + q3)*cos(q1)*(cos(q1)^2 + sin(q1)^2) + I(3,2,3)*cos(q2 + q3)*cos(q1)*(cos(q1)^2 + sin(q1)^2)) - 2*m3*(cm3(2)*cos(q2 + q3) + cm3(1)*sin(q2 + q3))*(cm3(1)*cos(q2 + q3) - cm3(2)*sin(q2 + q3)) + 2*m3*cos(q1)^2*(cm3(2)*cos(q2 + q3) + cm3(1)*sin(q2 + q3))*(cm3(1)*cos(q2 + q3) - cm3(2)*sin(q2 + q3)) + 2*m3*sin(q1)^2*(cm3(2)*cos(q2 + q3) + cm3(1)*sin(q2 + q3))*(cm3(1)*cos(q2 + q3) - cm3(2)*sin(q2 + q3))) + 0.5000*q1d*(sin(q1)*(cos(q2 + q3)*cos(q1)*(I(2,2,3)*cos(q2 + q3) + I(1,2,3)*sin(q2 + q3)) - cos(q2 + q3)*cos(q1)*(I(1,1,3)*cos(q2 + q3) - I(2,1,3)*sin(q2 + q3)) - sin(q1)*(I(1,3,3)*cos(q2 + q3) - I(2,3,3)*sin(q2 + q3)) + sin(q2 + q3)*cos(q1)*(I(2,1,3)*cos(q2 + q3) + I(1,1,3)*sin(q2 + q3)) + sin(q2 + q3)*cos(q1)*(I(1,2,3)*cos(q2 + q3) - I(2,2,3)*sin(q2 + q3))) - cos(q1)*(cos(q1)*(I(1,3,3)*cos(q2 + q3) - I(2,3,3)*sin(q2 + q3)) + sin(q2 + q3)*sin(q1)*(I(2,1,3)*cos(q2 + q3) + I(1,1,3)*sin(q2 + q3)) + sin(q2 + q3)*sin(q1)*(I(1,2,3)*cos(q2 + q3) - I(2,2,3)*sin(q2 + q3)) - cos(q2 + q3)*sin(q1)*(I(1,1,3)*cos(q2 + q3) - I(2,1,3)*sin(q2 + q3)) + cos(q2 + q3)*sin(q1)*(I(2,2,3)*cos(q2 + q3) + I(1,2,3)*sin(q2 + q3))) + I(3,1,3)*cos(q2 + q3)*(cos(q1)^2 + sin(q1)^2) - I(3,2,3)*sin(q2 + q3)*(cos(q1)^2 + sin(q1)^2))];
 
        
        

        Ct(1:3,1:3) =C;
        S =@(P) [ 0   -P(3)  P(2);
                P(3)  0    -P(1);
                -P(2)  P(1)   0];
        g0 = [0;0;-g];
        G = [                                                                                                0;
      - g*m3*(cm3(2)*sin(q2 + q3) - cm3(1)*cos(q2 + q3) + h2*sin(q2)) - g*m2*(cm2(2)*cos(q2) + cm2(1)*sin(q2));
                                                              g*m3*(cm3(1)*cos(q2 + q3) - cm3(2)*sin(q2 + q3))];
        Gt(1:3)= G;
        u = (Mt(1:3,1:3)*qdd(1:3)) + (Ct(1:3,1:3)*qd(1:3)) +Gt(1:3);
%         u = (Mt(1:3,1:3)*qdd(1:3)) + (Ct(1:3,1:3)*qd(1:3));
        ut(1:3)=u;
